simulink model "supply_demand_campus"  (Simulink 8.1)
settings: Solver=FixedStepDiscrete  StartTime=0.0  StopTime=Inf  FixedStep=60  RelTol=1e-3
libraries: CampusEnergyModeling x3
settings Model: Creator=wbernal  LastModifiedBy=wbernal
settings DebuggingCC: FcnCallInpInsideContextMsg=EnableAllAsWarning

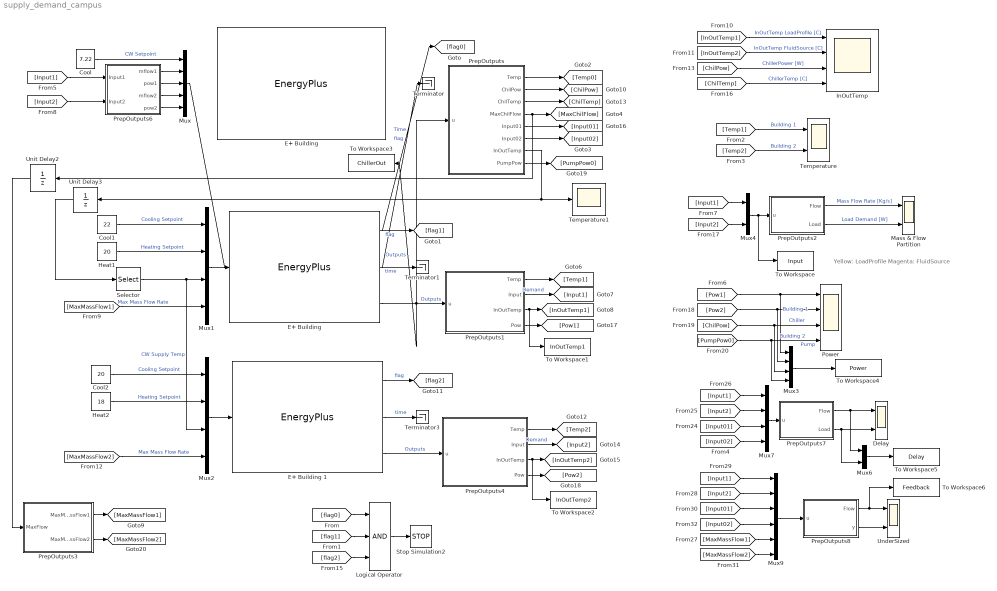
== system supply_demand_campus ==
  note: Yellow: LoadProfile
      | Magenta: FluidSource
  Cool : Constant  Value=7.22
  Cool1 : Constant  Value=22
  Cool2 : Constant  Value=20
  Delay : Scope  NumInputPorts=2
      settings: TickLabels=on  TimeRange=450000  YMin=0~-23000  YMax=2~0  SaveName=ScopeData8
  E+ Building : CampusEnergyModeling/Buildings/EnergyPlus  progname='C:\EnergyPlusV8-0-0\RunEPlus.bat'  modelfile=[pwd '\Building1\5ZoneAirCool']  weatherfile='USA_CO_Golden-NREL.724666_TMY3'  workdir=[pwd '\Building1']  timeout=6000  port=0  host=''  bcvtbdir=''  deltaT=60  noutputd=13
  E+ Building 1 : CampusEnergyModeling/Buildings/EnergyPlus  progname='C:\EnergyPlusV8-0-0\RunEPlus.bat'  modelfile=[pwd '\Building2\5ZoneAirCool']  weatherfile='USA_CO_Golden-NREL.724666_TMY3'  workdir=[pwd '\Building2']  timeout=6000  port=0  host=''  bcvtbdir=''  deltaT=60  noutputd=13
  E+ Building : CampusEnergyModeling/Buildings/EnergyPlus  progname='C:\EnergyPlusV8-0-0\RunEPlus.bat'  modelfile=[pwd '\ElectricChiller\ElectricChiller']  weatherfile='USA_CO_Golden-NREL.724666_TMY3'  workdir=[pwd '\ElectricChiller']  timeout=6000  port=0  host=''  bcvtbdir=''  deltaT=60  noutputd=13
  Heat1 : Constant  Value=20
  Heat2 : Constant  Value=18
  InOutTemp : Scope  NumInputPorts=4
      settings: TimeRange=450000  YMin=0~0~0~7  YMax=15~14~12000~11.5  SaveName=ScopeData3
  Logical Operator : Logic  Inputs=3  IconShape=distinctive  AllPortsSameDT=off  OutDataTypeStr=boolean
  Mass & Flow Partition : Scope  NumInputPorts=2
      settings: TickLabels=on  TimeRange=450000  YMin=0~-0  YMax=2.2~47500  SaveName=ScopeData2
  Mux : Mux  Inputs=5
  Mux{1..3,7} (4 alike) : Mux
  Mux4 : Mux  Inputs=2
  Mux6 : Mux  Inputs=2
  Mux9 : Mux  Inputs=6
  Power : Scope  NumInputPorts=4
      settings: TimeRange=450000  YMin=12~12~-5~-5  YMax=32~32~5~5
  PrepOutputs : MATLAB Function  TreatAsAtomicUnit=on
  PrepOutputs1 : MATLAB Function  TreatAsAtomicUnit=on
  PrepOutputs2 : MATLAB Function  TreatAsAtomicUnit=on
  PrepOutputs3 : MATLAB Function  TreatAsAtomicUnit=on
  PrepOutputs4 : MATLAB Function  Priority=2  TreatAsAtomicUnit=on
  PrepOutputs6 : MATLAB Function  TreatAsAtomicUnit=on
  PrepOutputs7 : MATLAB Function  TreatAsAtomicUnit=on
  PrepOutputs8 : MATLAB Function  TreatAsAtomicUnit=on
  Selector : Selector  InputPortWidth=4  IndexOptions=Index vector (dialog)  Indices=[1]  OutputSizes=1
  Stop Simulation2 : Stop
  Temperature : Scope  NumInputPorts=2
      settings: TimeRange=450000  YMin=12~12  YMax=32~32
  Temperature1 : Scope
      settings: TimeRange=450000  YMin=12  YMax=32  SaveName=ScopeData6
  Terminator : Terminator
  Terminator1 : Terminator
  Terminator3 : Terminator
  To Workspace : ToWorkspace  VariableName=Input  SampleTime=-1  SaveFormat=Structure With Time
  To Workspace1 : ToWorkspace  VariableName=InOutTemp1  SampleTime=-1  SaveFormat=Structure With Time
  To Workspace2 : ToWorkspace  VariableName=InOutTemp2  SampleTime=-1  SaveFormat=Structure With Time
  To Workspace3 : ToWorkspace  VariableName=ChillerOut  SampleTime=-1  SaveFormat=Structure With Time
  To Workspace4 : ToWorkspace  VariableName=Power  SampleTime=-1  SaveFormat=Structure With Time
  To Workspace5 : ToWorkspace  VariableName=Delay  SampleTime=-1  SaveFormat=Structure With Time
  To Workspace6 : ToWorkspace  VariableName=Feedback  SampleTime=-1  SaveFormat=Structure With Time
  UnderSized : Scope  NumInputPorts=2
      settings: TickLabels=on  TimeRange=450000  YMin=0~0  YMax=2~2  SaveName=ScopeData9
  Unit Delay2 : UnitDelay  SampleTime=-1
  Unit Delay3 : UnitDelay  SampleTime=-1
  wires:
  E+ Building/1 -> [flag0]  "flag"
  Cool/1 -> Mux/1  "CW Setpoint"
  Mux/1 -> E+ Building/1
  Cool1/1 -> Mux1/1  "Cooling Setpoint"
  Heat1/1 -> Mux1/2  "Heating Setpoint"
  Mux1/1 -> E+ Building/1
  E+ Building/1 -> [flag1]  "flag"
  Logical Operator/1 -> Stop Simulation2/1
  [flag0] -> Logical Operator/1
  [flag1] -> Logical Operator/2
  E+ Building/2 -> Terminator/1  "Time"
  E+ Building/2 -> Terminator1/1  "time"
  E+ Building/3 -> To Workspace3/1, PrepOutputs/1(u)  "Outputs"
  E+ Building/3 -> PrepOutputs1/1(u)  "Outputs"
  PrepOutputs1/1(Temp) -> [Temp1]
  PrepOutputs1/2(Input) -> [Input1]  "Demand"
  PrepOutputs1/3(InOutTemp) -> [InOutTemp1], To Workspace1/1
  [Temp1] -> Temperature/1  "Building 1"
  [Temp2] -> Temperature/2  "Building 2"
  Mux4/1 -> PrepOutputs2/1(u), To Workspace/1
  PrepOutputs2/1(Flow) -> Mass & Flow Partition/1  "Mass Flow Rate [Kg/s]"
  PrepOutputs2/2(Load) -> Mass & Flow Partition/2  "Load Demand [W]"
  [InOutTemp1] -> InOutTemp/1  "InOutTemp LoadProfile [C]"
  [InOutTemp2] -> InOutTemp/2  "InOutTemp FluidSource [C]"
  [MaxMassFlow1] -> Mux1/4  "Max Mass Flow Rate"
  [ChilPow] -> InOutTemp/3  "ChillerPower [W]"
  [ChilTemp] -> InOutTemp/4  "ChillerTemp [C]"
  PrepOutputs3/1(MaxMassFlow1) -> [MaxMassFlow1]
  Cool2/1 -> Mux2/1  "Cooling Setpoint"
  Heat2/1 -> Mux2/2  "Heating Setpoint"
  Mux2/1 -> E+ Building 1/1
  E+ Building 1/1 -> [flag2]  "flag"
  E+ Building 1/2 -> Terminator3/1  "time"
  E+ Building 1/3 -> PrepOutputs4/1(u)  "Outputs"
  PrepOutputs4/1(Temp) -> [Temp2]
  PrepOutputs4/2(Input) -> [Input2]  "Demand"
  PrepOutputs4/3(InOutTemp) -> [InOutTemp2], To Workspace2/1
  [MaxMassFlow2] -> Mux2/4  "Max Mass Flow Rate"
  [flag2] -> Logical Operator/3
  PrepOutputs/1(Temp) -> [Temp0]
  PrepOutputs/2(ChilPow) -> [ChilPow]
  PrepOutputs/3(ChilTemp) -> [ChilTemp]
  PrepOutputs/5(Input01) -> [Input01]
  PrepOutputs/6(Input02) -> [Input02]
  [Input1] -> Mux4/1
  [Input2] -> Mux4/2
  PrepOutputs1/4(Pow) -> [Pow1]
  PrepOutputs4/4(Pow) -> [Pow2]
  [Pow2] -> Power/2, Mux3/2  "Building 2"
  [ChilPow] -> Power/3, Mux3/3  "Chiller"
  [Pow1] -> Power/1, Mux3/1  "Building 1"
  PrepOutputs/8(PumpPow) -> [PumpPow0]
  [PumpPow0] -> Power/4, Mux3/4  "Pump"
  Mux3/1 -> To Workspace4/1
  Selector/1 -> Mux1/3, Mux2/3  "CW Supply Temp"
  PrepOutputs3/2(MaxMassFlow2) -> [MaxMassFlow2]
  [Input02] -> Mux7/4
  [Input1] -> Mux7/1
  [Input2] -> Mux7/2
  [Input01] -> Mux7/3
  Mux7/1 -> PrepOutputs7/1(u)
  PrepOutputs7/1(Flow) -> Delay/1, Mux6/1
  PrepOutputs7/2(Load) -> Delay/2, Mux6/2
  Mux6/1 -> To Workspace5/1
  [Input1] -> Mux9/1
  [Input2] -> Mux9/2
  Mux9/1 -> PrepOutputs8/1(u)
  PrepOutputs8/1(Flow) -> UnderSized/1, To Workspace6/1
  [Input01] -> Mux9/3
  [Input02] -> Mux9/4
  [MaxMassFlow1] -> Mux9/5
  [MaxMassFlow2] -> Mux9/6
  PrepOutputs8/2(y) -> UnderSized/2
  PrepOutputs/7(InOutTemp) -> Unit Delay3/1, Temperature1/1
  PrepOutputs/4(MaxChilFlow) -> [MaxChilFlow], Unit Delay2/1
  PrepOutputs6/1(mflow1) -> Mux/2
  PrepOutputs6/2(pow1) -> Mux/3
  PrepOutputs6/3(mflow2) -> Mux/4
  PrepOutputs6/4(pow2) -> Mux/5
  [Input1] -> PrepOutputs6/1(Input1)
  [Input2] -> PrepOutputs6/2(Input2)
  Unit Delay2/1 -> PrepOutputs3/1(MaxFlow)
  Unit Delay3/1 -> Selector/1

== matlab function PrepOutputs1 ==
  data: u input double; Temp output double; Input output double; InOutTemp output double; Pow output double
function [Temp,Input,InOutTemp, Pow] = fcn(u)

Temp = u(1:7);          % Out, Room Temp
Input = u(8:9);         % Flow Rate, Load 
InOutTemp = u(10:11);   % Inlet/Outlet Water Temperature
Pow = u(12:13);         % Power

== matlab function PrepOutputs ==
  data: u input double; Temp output double; ChilPow output double; ChilTemp output double; MaxChilFlow output double; Input01 output double; Input02 output double; InOutTemp output double; PumpPow output double
function [Temp,ChilPow,ChilTemp, MaxChilFlow, Input01, Input02, InOutTemp, PumpPow] = fcn(u)

Temp = u(1);        % Temperature(Outdoor, Zones)
ChilPow = u(2);     % Chiller Power
ChilTemp = u(3);    % Chiller Water Temperature
MaxChilFlow = u(4); % Maximum Chiller Flow 
Input01 = u(5:6);   % Mass Flow Rate and Power Load 
Input02 = u(7:8);   % Mass Flow Rate and Power Load
InOutTemp = u(9:12);% Inlet/Outlet Water Temperature   
PumpPow = u(13);    % Pump Power

== matlab function PrepOutputs2 ==
  data: Flow output double; u input double; Load output double
function [Flow, Load] = fcn(u)
% u contains 
% Input1 - Chilller
%   MassFlowRate
%   Load Demand
% Input2 - Building
%   MassFlowRate
%   Load Demand
Flow = [u(1) u(3) u(1)+u(3)];
Load = [-u(2) -u(4) -u(2)-u(4)];

== matlab function PrepOutputs3 ==
  data: MaxMassFlow1 output double; MaxFlow input double; MaxMassFlow2 output double
function [MaxMassFlow1, MaxMassFlow2] = fcn(MaxFlow)
% Transform into [Kg/s] Split Evenly
MaxFlow = MaxFlow*1000;
%if Input1+Input2 > MaxFlow
MaxMassFlow1 = MaxFlow/2;
MaxMassFlow2 = MaxFlow/2;
%else
%    MaxMassFlow1 =  
%    MaxMassFlow2 = MaxFlow - Input;
%end

== matlab function PrepOutputs4 ==
  data: u input double; Temp output double; Input output double; InOutTemp output double; Pow output double
function [Temp,Input,InOutTemp,Pow] = fcn(u)

Temp = u(1:7);          % Out, Room Temp
Input = u(8:9);         % Flow Rate, Load 
InOutTemp = u(10:11);   % Inlet/Outlet Water Temperature
Pow = u(12:13);         % Total Power

== matlab function PrepOutputs6 ==
  data: Input1 input double; Input2 input double; mflow1 output double; pow1 output double; mflow2 output double; pow2 output double
function [mflow1, pow1, mflow2, pow2] = fcn(Input1, Input2)
ratio = 0.005;
mflow1 = Input1(1)/ratio/1000;
pow1 = Input1(2);
mflow2 = Input2(1)/ratio/1000; 
pow2 = Input2(2);

== matlab function PrepOutputs7 ==
  data: Flow output double; u input double; Load output double
function [Flow, Load] = fcn(u)
% u contains 
% Input1 - Chilller
%   MassFlowRate
%   Load Demand
% Input2 - Building
%   MassFlowRate
%   Load Demand
Flow = [u(1) u(5)];
Load = [u(2) u(6)];

== matlab function PrepOutputs8 ==
  data: Flow output double; u input double; y output double
function [Flow, y]  = fcn(u)
% u contains 
% Input1 - Chilller
%   MassFlowRate
%   Load Demand
% Input2 - Building
%   MassFlowRate
%   Load Demand
Flow = [u(1) u(5) u(9)];
y  = [u(3) u(7) u(10)];
